simulink model "control_main"  (R2026a)
settings: Solver=VariableStepAuto  StopTime=inf
InitFcn:
  | load(fullfile('calibration_data','sensor_calibration.mat'),'coefficients');
  | load(fullfile('calibration_data','pump_calibration.mat'),'Q');
  | load(fullfile('calibration_data','az_calibration.mat'),'az');
  | 
  | actuallevel1 = 200;
values from neighbouring files (symbols this model uses):
  coefficients = [20.111978783 20.2762923351 20.4770477048]    [sensor_calibration.mat]
  sensor_low = [1.00893772894 1.03633699634 1.00974358974]    [sensor_calibration.mat]
undefined symbols (not defined in the file or in its folder): az, Q
libraries: instrumentseriallib x3
settings Model: Creator=user  LastModifiedBy=jinyu

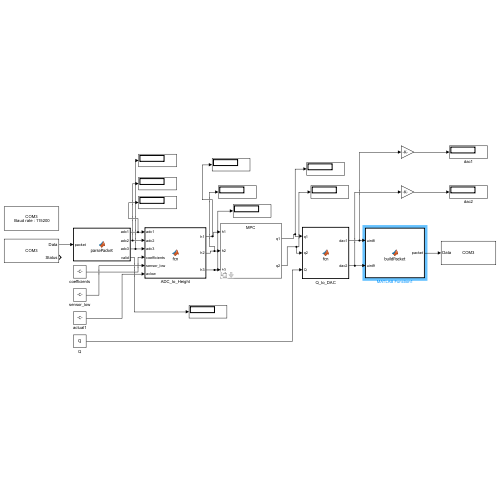
[thumbnail: Simulink's stored preview of the top-level diagram]
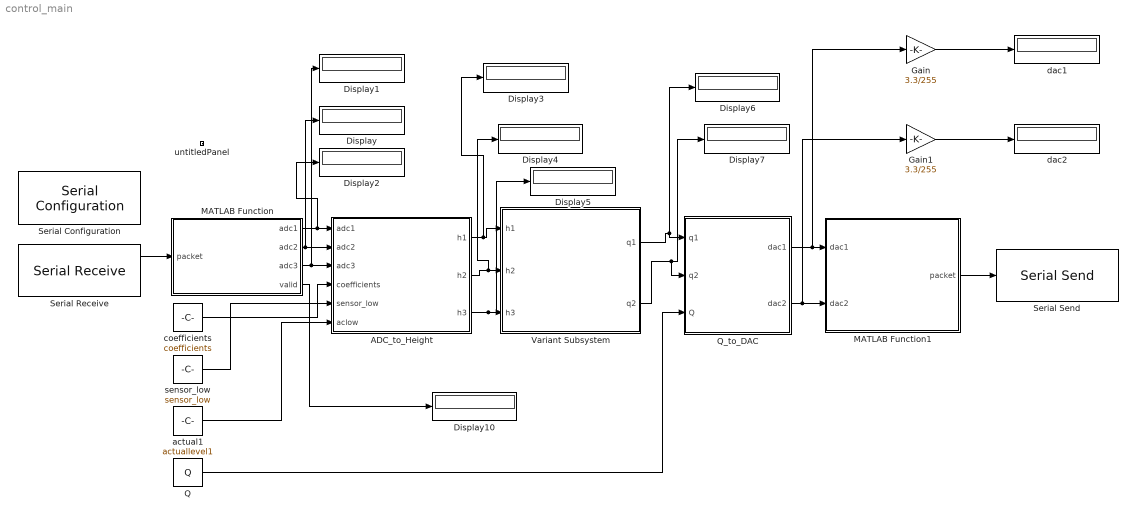
== system control_main ==
  ADC_to_Height : MATLAB Function  TreatAsAtomicUnit=on
  Display{,1..7,10} (9 alike) : Display
  Gain : Gain  Gain=3.3/255
  Gain1 : Gain  Gain=3.3/255
  MATLAB Function : MATLAB Function  TreatAsAtomicUnit=on
  MATLAB Function1 : MATLAB Function  TreatAsAtomicUnit=on
  Q : Constant  Value=Q
  Q_to_DAC : MATLAB Function  TreatAsAtomicUnit=on
  Serial Configuration : instrumentseriallib/Serial Configuration  Priority=-200000  PortSel=COM3  Port=COM3  ComPort=COM3  BaudRate=115200  DataBits=8  Parity=none  StopBits=1  ByteOrder=little-endian  FlowControl=none  Timeout=10  SimulateUsing=Interpreted execution  BlockInModel=on  aMode=1
  Serial Receive : instrumentseriallib/Serial Receive  Priority=1  PortSel=COM3  Port=COM3  ComPort=COM3  DataType=uint8  SaveDataType=uint8  ToggleHeader=on  Header=[0xAA 0x01]  ToggleDataSize=on  DataSize=[7]  ToggleTerminator=off  Terminator=<none>  CustomTerminator=[]  InputFormat=Column major  EnableBlockingMode=off  ActionDataUnavailable=Output last received value  ActionWhenDataUnavailable=Output last received value  CustomValue=0  SampleTime=0.01  SimulateUsing=Interpreted execution  BlockInModel=on  aMode=1  LibraryInUse=instrumentlib
  Serial Send : instrumentseriallib/Serial Send  Priority=1  PortSel=COM3  Port=COM3  ComPort=COM3  Header=[]  Terminator=<none>  CustomTerminator=[]  EnableBlockingMode=off  SimulateUsing=Interpreted execution  BlockInModel=on  aMode=1
  Variant Subsystem : Subsystem  Variant=on  mask{ctrl_mode=MPC, r1=300, r2=150, r3=200, Kp_PI=1, Ki_PI=1, Kp1_PI=1, Ki1_PI=1, Kp2_PI=1, Ki2_PI=1, Kp_IO=1, Kp1_IO=1, Kp3_IO=1, Kd3_IO=1, K_BS=1, Kz_BS=1, K1_BS=1, K3_BS=1, S1=0.05, S2=0.05, S3=20, R1_MPC=0.05, R2_MPC=0.05, H=15}
      mask prompts: r1 "Tank1"; r2 "Tank2"; r3 "Tank3"; Kp_PI "Kp"; Ki_PI "Ki"; Kp1_PI "Kp1"; Ki1_PI "Ki1"; Kp2_PI "Kp2"; Ki2_PI "Ki2"; Kp_IO "Kp"; Kp1_IO "Kp1"; Kp3_IO "Kp3"; Kd3_IO "Kd3"; K_BS "K"; Kz_BS "Kz"; K1_BS "K1"; K3_BS "K3"; R1_MPC "R1"; R2_MPC "R2"
      mask DialogControl ParameterGroupVar Prompt: Controller
      mask DialogControl Container4 Prompt: Reference Levels
      mask DialogControl Container5 Prompt: PI SISO Parameters
      mask DialogControl Container6 Prompt: PI MIMO Parameters
      mask DialogControl Container7 Prompt: IO Linearization SISO
      mask DialogControl Container8 Prompt: IO Linearization MIMO
      mask DialogControl Container9 Prompt: Backstepping SISO
      mask DialogControl Container10 Prompt: Backstepping MIMO
      mask DialogControl Container11 Prompt: MPC
  actual1 : Constant  Value=actuallevel1
  coefficients : Constant  Value=coefficients
  dac1 : Display
  dac2 : Display
  sensor_low : Constant  Value=sensor_low
  untitledPanel : Subsystem  Tag=HiddenForWebPanel  IsWebBlockPanel=on
  wires:
  MATLAB Function1/1(packet) -> Serial Send/1
  Serial Receive/1 -> MATLAB Function/1(packet)
  MATLAB Function/2(adc2) -> ADC_to_Height/2(adc2), Display/1
  MATLAB Function/3(adc3) -> ADC_to_Height/3(adc3), Display1/1
  coefficients/1 -> ADC_to_Height/4(coefficients)
  sensor_low/1 -> ADC_to_Height/5(sensor_low)
  actual1/1 -> ADC_to_Height/6(aclow)
  Q_to_DAC/1(dac1) -> Gain/1, MATLAB Function1/1(dac1)
  Q_to_DAC/2(dac2) -> Gain1/1, MATLAB Function1/2(dac2)
  Q/1 -> Q_to_DAC/3(Q)
  ADC_to_Height/1(h1) -> Display3/1, Variant Subsystem/1(h1)
  ADC_to_Height/2(h2) -> Display4/1, Variant Subsystem/2(h2)
  ADC_to_Height/3(h3) -> Display5/1, Variant Subsystem/3(h3)
  Variant Subsystem/1(q1) -> Display6/1, Q_to_DAC/1(q1)
  Variant Subsystem/2(q2) -> Display7/1, Q_to_DAC/2(q2)
  MATLAB Function/1(adc1) -> ADC_to_Height/1(adc1), Display2/1
  MATLAB Function/4(valid) -> Display10/1
  Gain/1 -> dac1/1
  Gain1/1 -> dac2/1

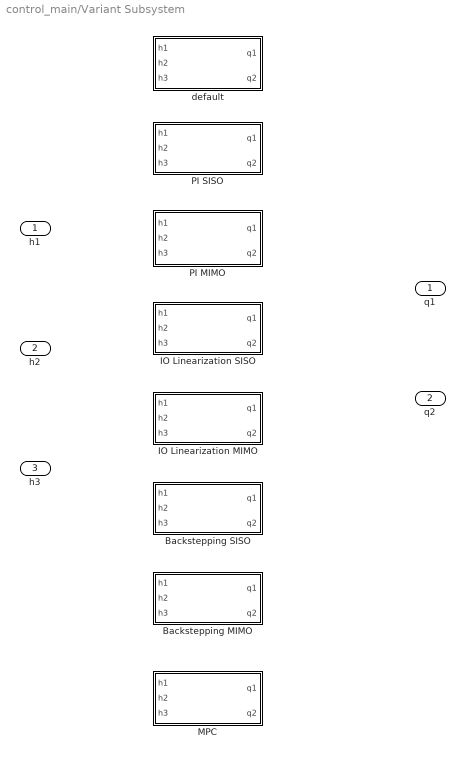
== system control_main/Variant Subsystem ==
  h1 : Inport
  h2 : Inport  Port=2
  h3 : Inport  Port=3
  Backstepping MIMO : Subsystem  VariantControl=ctrl_mode == 6
  Backstepping SISO : Subsystem  VariantControl=ctrl_mode == 5
  IO Linearization MIMO : Subsystem  VariantControl=ctrl_mode == 4
  IO Linearization SISO : Subsystem  VariantControl=ctrl_mode == 3
  MPC : Subsystem  VariantControl=ctrl_mode == 7
  PI MIMO : Subsystem  VariantControl=ctrl_mode == 2
  PI SISO : Subsystem  VariantControl=ctrl_mode == 1
  default : Subsystem  VariantControl=ctrl_mode == 0
  q1 : Outport
  q2 : Outport  Port=2

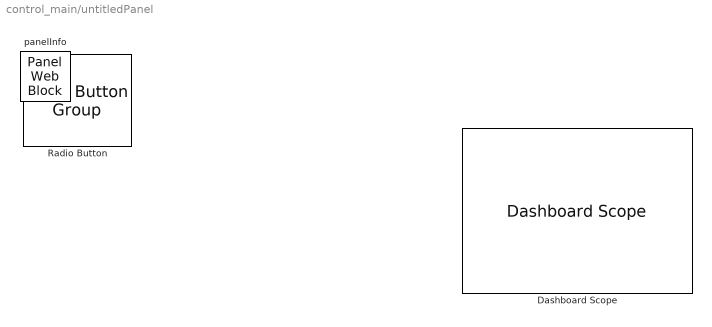
== system control_main/untitledPanel ==
  Dashboard Scope : DashboardScope  Tag=HiddenForWebPanel  PanelInfo="{\"height\":404,\"left\":393,\"panelId\":\"panelId-8aad0df7-f305-4620-9adc-6ae666dad641\",\"top\":27,\"type\":\"panelChild\",\"version\":\"2019b\",\"width\":464,\"zIndex\":1500004}"  Ymin=50  Ymax=550  FontColor=[0.0, 0.0, 0.0]
  Radio Button : RadioButtonGroup  Tag=HiddenForWebPanel  PanelInfo="{\"height\":384,\"left\":33,\"panelId\":\"panelId-8aad0df7-f305-4620-9adc-6ae666dad641\",\"top\":42,\"type\":\"panelChild\",\"version\":\"2019b\",\"width\":318,\"zIndex\":1500002}"  ButtonGroupName=Control Mode
  panelInfo : PanelWebBlock  Tag=HiddenForWebPanel  PanelInfo="{\"compacted\":true,\"height\":468,\"isActiveTab\":true,\"left\":782,\"name\":\"Panel\",\"panelId\":\"panelId-8aad0df7-f305-4620-9adc-6ae666dad641\",\"tabIndex\":0,\"tabbedSetId\":\"tabbedSet3175960063\",\"top\":92,\"type\":\"panel\",\"version\":\"2019b\",\"visible\":true,\"width\":881,\"zIndex\":1500002}"  PanelSnapshot=<binary blob, 100836 chars, not shown>

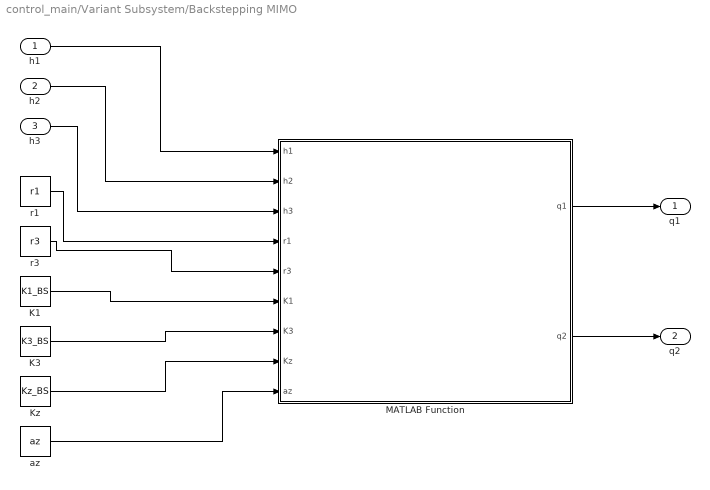
== system control_main/Variant Subsystem/Backstepping MIMO ==
  h1 : Inport
  h2 : Inport  Port=2
  h3 : Inport  Port=3
  K1 : Constant  Value=K1_BS
  K3 : Constant  Value=K3_BS
  Kz : Constant  Value=Kz_BS
  MATLAB Function : MATLAB Function  TreatAsAtomicUnit=on
  az : Constant  Value=az
  r1 : Constant  Value=r1
  r3 : Constant  Value=r3
  q1 : Outport
  q2 : Outport  Port=2
  wires:
  MATLAB Function/1(q1) -> q1/1
  MATLAB Function/2(q2) -> q2/1
  h1/1 -> MATLAB Function/1(h1)
  h2/1 -> MATLAB Function/2(h2)
  h3/1 -> MATLAB Function/3(h3)
  r1/1 -> MATLAB Function/4(r1)
  r3/1 -> MATLAB Function/5(r3)
  K1/1 -> MATLAB Function/6(K1)
  K3/1 -> MATLAB Function/7(K3)
  Kz/1 -> MATLAB Function/8(Kz)
  az/1 -> MATLAB Function/9(az)

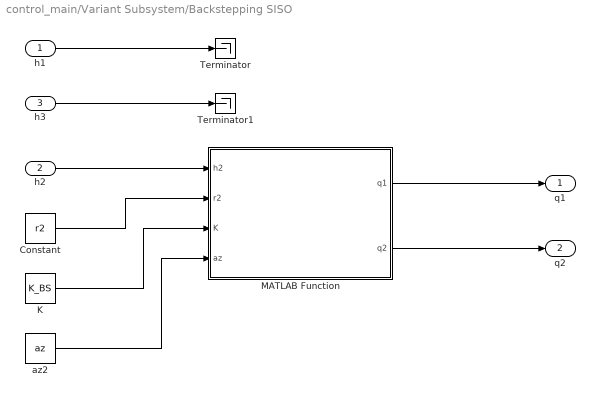
== system control_main/Variant Subsystem/Backstepping SISO ==
  h1 : Inport
  h2 : Inport  Port=2
  h3 : Inport  Port=3
  Constant : Constant  Value=r2
  K : Constant  Value=K_BS
  MATLAB Function : MATLAB Function  TreatAsAtomicUnit=on
  Terminator : Terminator
  Terminator1 : Terminator
  az2 : Constant  Value=az
  q1 : Outport
  q2 : Outport  Port=2
  wires:
  Constant/1 -> MATLAB Function/2(r2)
  az2/1 -> MATLAB Function/4(az)
  MATLAB Function/1(q1) -> q1/1
  MATLAB Function/2(q2) -> q2/1
  K/1 -> MATLAB Function/3(K)
  h3/1 -> Terminator1/1
  h2/1 -> MATLAB Function/1(h2)
  h1/1 -> Terminator/1

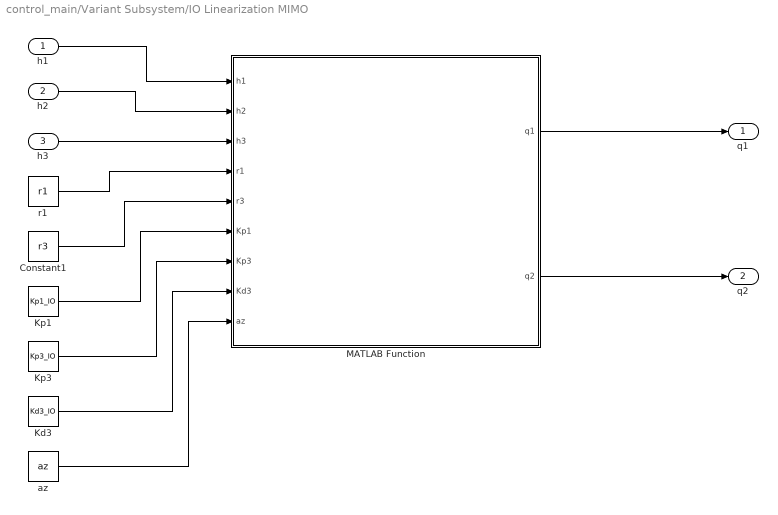
== system control_main/Variant Subsystem/IO Linearization MIMO ==
  h1 : Inport
  h2 : Inport  Port=2
  h3 : Inport  Port=3
  Constant1 : Constant  Value=r3
  Kd3 : Constant  Value=Kd3_IO
  Kp1 : Constant  Value=Kp1_IO
  Kp3 : Constant  Value=Kp3_IO
  MATLAB Function : MATLAB Function  TreatAsAtomicUnit=on
  az : Constant  Value=az
  r1 : Constant  Value=r1
  q1 : Outport
  q2 : Outport  Port=2
  wires:
  h2/1 -> MATLAB Function/2(h2)
  MATLAB Function/2(q2) -> q2/1
  MATLAB Function/1(q1) -> q1/1
  h1/1 -> MATLAB Function/1(h1)
  h3/1 -> MATLAB Function/3(h3)
  r1/1 -> MATLAB Function/4(r1)
  Constant1/1 -> MATLAB Function/5(r3)
  Kp1/1 -> MATLAB Function/6(Kp1)
  Kp3/1 -> MATLAB Function/7(Kp3)
  Kd3/1 -> MATLAB Function/8(Kd3)
  az/1 -> MATLAB Function/9(az)

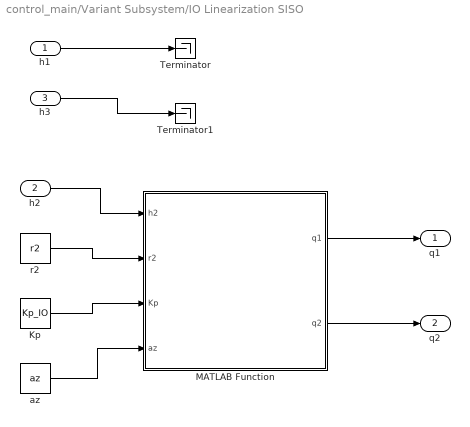
== system control_main/Variant Subsystem/IO Linearization SISO ==
  h1 : Inport
  h2 : Inport  Port=2
  h3 : Inport  Port=3
  Kp : Constant  Value=Kp_IO
  MATLAB Function : MATLAB Function  TreatAsAtomicUnit=on
  Terminator : Terminator
  Terminator1 : Terminator
  az : Constant  Value=az
  r2 : Constant  Value=r2
  q1 : Outport
  q2 : Outport  Port=2
  wires:
  h2/1 -> MATLAB Function/1(h2)
  r2/1 -> MATLAB Function/2(r2)
  Kp/1 -> MATLAB Function/3(Kp)
  MATLAB Function/1(q1) -> q1/1
  MATLAB Function/2(q2) -> q2/1
  az/1 -> MATLAB Function/4(az)
  h1/1 -> Terminator/1
  h3/1 -> Terminator1/1

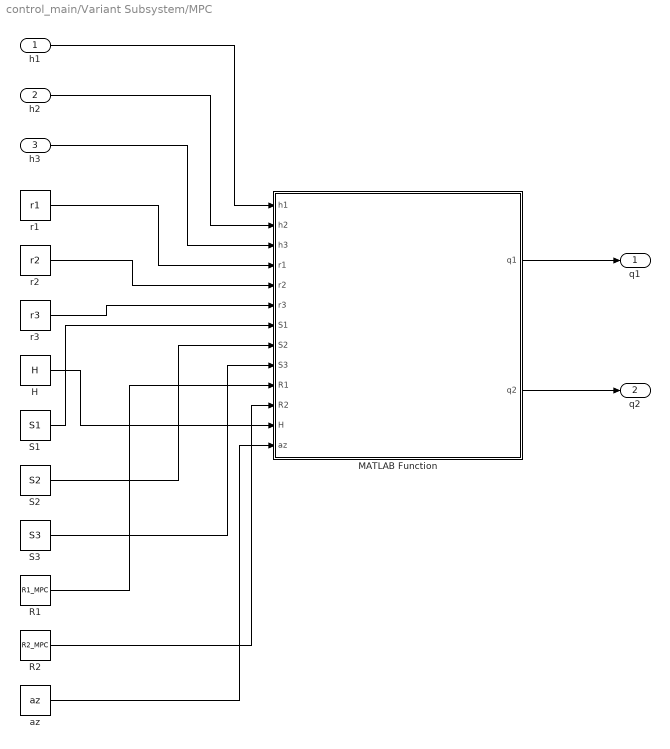
== system control_main/Variant Subsystem/MPC ==
  h1 : Inport
  h2 : Inport  Port=2
  h3 : Inport  Port=3
  H : Constant  Value=H
  MATLAB Function : MATLAB Function  TreatAsAtomicUnit=on
  R1 : Constant  Value=R1_MPC
  R2 : Constant  Value=R2_MPC
  S1 : Constant  Value=S1
  S2 : Constant  Value=S2
  S3 : Constant  Value=S3
  az : Constant  Value=az
  r1 : Constant  Value=r1
  r2 : Constant  Value=r2
  r3 : Constant  Value=r3
  q1 : Outport
  q2 : Outport  Port=2
  wires:
  MATLAB Function/1(q1) -> q1/1
  MATLAB Function/2(q2) -> q2/1
  h1/1 -> MATLAB Function/1(h1)
  h2/1 -> MATLAB Function/2(h2)
  h3/1 -> MATLAB Function/3(h3)
  r1/1 -> MATLAB Function/4(r1)
  r2/1 -> MATLAB Function/5(r2)
  r3/1 -> MATLAB Function/6(r3)
  H/1 -> MATLAB Function/12(H)
  S1/1 -> MATLAB Function/7(S1)
  S2/1 -> MATLAB Function/8(S2)
  S3/1 -> MATLAB Function/9(S3)
  R1/1 -> MATLAB Function/10(R1)
  R2/1 -> MATLAB Function/11(R2)
  az/1 -> MATLAB Function/13(az)

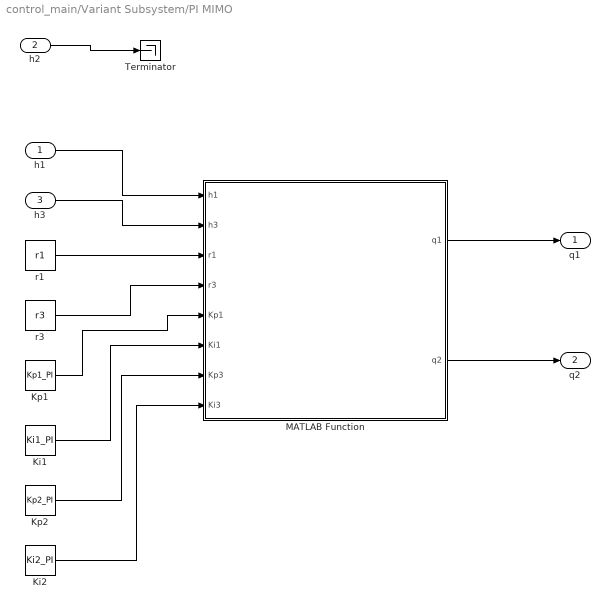
== system control_main/Variant Subsystem/PI MIMO ==
  h1 : Inport
  h2 : Inport  Port=2
  h3 : Inport  Port=3
  Ki1 : Constant  Value=Ki1_PI
  Ki2 : Constant  Value=Ki2_PI
  Kp1 : Constant  Value=Kp1_PI
  Kp2 : Constant  Value=Kp2_PI
  MATLAB Function : MATLAB Function  TreatAsAtomicUnit=on
  Terminator : Terminator
  r1 : Constant  Value=r1
  r3 : Constant  Value=r3
  q1 : Outport
  q2 : Outport  Port=2
  wires:
  MATLAB Function/2(q2) -> q2/1
  MATLAB Function/1(q1) -> q1/1
  h1/1 -> MATLAB Function/1(h1)
  h3/1 -> MATLAB Function/2(h3)
  r1/1 -> MATLAB Function/3(r1)
  r3/1 -> MATLAB Function/4(r3)
  Kp1/1 -> MATLAB Function/5(Kp1)
  Ki1/1 -> MATLAB Function/6(Ki1)
  Kp2/1 -> MATLAB Function/7(Kp3)
  Ki2/1 -> MATLAB Function/8(Ki3)
  h2/1 -> Terminator/1

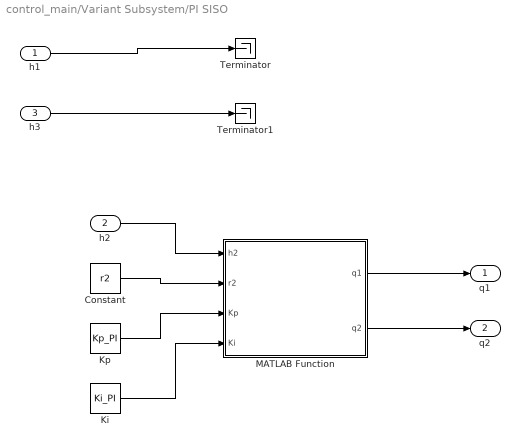
== system control_main/Variant Subsystem/PI SISO ==
  h1 : Inport
  h2 : Inport  Port=2
  h3 : Inport  Port=3
  Constant : Constant  Value=r2
  Ki : Constant  Value=Ki_PI
  Kp : Constant  Value=Kp_PI
  MATLAB Function : MATLAB Function  TreatAsAtomicUnit=on
  Terminator : Terminator
  Terminator1 : Terminator
  q1 : Outport
  q2 : Outport  Port=2
  wires:
  MATLAB Function/2(q2) -> q2/1
  MATLAB Function/1(q1) -> q1/1
  h2/1 -> MATLAB Function/1(h2)
  Constant/1 -> MATLAB Function/2(r2)
  Kp/1 -> MATLAB Function/3(Kp)
  Ki/1 -> MATLAB Function/4(Ki)
  h1/1 -> Terminator/1
  h3/1 -> Terminator1/1

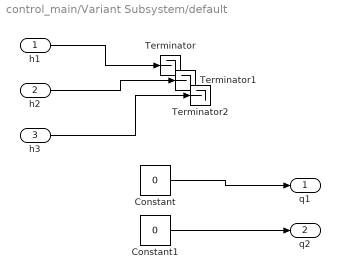
== system control_main/Variant Subsystem/default ==
  h1 : Inport
  h2 : Inport  Port=2
  h3 : Inport  Port=3
  Constant : Constant  Value=0
  Constant1 : Constant  Value=0
  Terminator : Terminator
  Terminator1 : Terminator
  Terminator2 : Terminator
  q1 : Outport
  q2 : Outport  Port=2
  wires:
  Constant/1 -> q1/1
  Constant1/1 -> q2/1
  h1/1 -> Terminator/1
  h2/1 -> Terminator1/1
  h3/1 -> Terminator2/1

== matlab function control_main/Variant Subsystem/IO Linearization MIMO/MATLAB Function ==
  data: h1 input; q1 output; h2 input; h3 input; r1 input; r3 input; Kp1 input; Kp3 input; Kd3 input; az input; q2 output
function [q1,q2] = IO_MIMO(h1,h2,h3,r1,r3,Kp1,Kp3,Kd3,az)
%对q13和q32分别求一阶和二阶导推q1q2表达式

A  = 154.0;
Sn = 0.5;
g  = 981.0;
TWOG = 2*g;

az1 = az(1);
az2 = az(2);
az3 = az(3);

q13 = az1 * Sn * sqrt(TWOG * abs(h1-h3));
q32 = az3 * Sn * sqrt(TWOG * abs(h3-h2));
q20 = az2 * Sn * sqrt(TWOG * max(h2,0));

e1 = r1 - h1;
q1 = A*Kp1*e1 + 2*q13 - q32;
q1 = min(max(q1,0),800);

den13 = sqrt(abs(h1-h3));
den32 = sqrt(abs(h3-h2));

if den13 < 1e-6
    den13 = 1e-6;
end

if den32 < 1e-6
    den32 = 1e-6;
end

k1 = az1 * den32 / (az3 * den13);
k2 = (TWOG * az3 * Sn) / (2 * sqrt(TWOG * abs(h3-h2) + 1e-6));

persistent e3_old

if isempty(e3_old)
    e3_old = 0;
end

Ts = 0.01;
e3 = r3 - h3;

pd = Kp3*e3 + Kd3*(e3 - e3_old)/Ts;

q2 = -k1*(q1 - 2*q13 + q32) ...
     + (q13 - 2*q32 + q20) ...
     + A*A*(1/k2)*pd;

q2 = min(max(q2,0),800);

e3_old = e3;

end

== matlab function control_main/Variant Subsystem/Backstepping SISO/MATLAB Function ==
  data: h2 input; q1 output; r2 input; K input; az input; q2 output
function [q1,q2] = Backstepping_SISO(h2,r2,K,az)
% backstepping误差指数减小  de/dt=-Ke​

A  = 154.0;
Sn = 0.5;
g  = 981.0;
Ofc2 = az(2);

q20 = Ofc2 * Sn * sqrt(2*g*max(h2,0));

q1 = 0;
q2 = q20 + A*K*(r2 - h2);

q2 = min(max(q2,0),800);

end

== matlab function control_main/Variant Subsystem/Backstepping MIMO/MATLAB Function ==
  data: h1 input; q1 output; h2 input; h3 input; r1 input; r3 input; K1 input; K3 input; Kz input; az input; q2 output
function [q1,q2] = Backstepping_MIMO(h1,h2,h3,r1,r3,K1,K3,Kz,az)
% Backstepping MIMO for Tank1 and Tank3
% K1       : Tank1 error gain
% K3       : Tank3 virtual control gain
% Kz       : q32 tracking gain


A  = 154.0;
Sn = 0.5;
g  = 981.0;
TWOG = 2*g;
epsv = 1e-6;

az1 = az(1);
az2 = az(2);
az3 = az(3);

q13 = az1 * Sn * sqrt(TWOG * max(h1-h3, 0));
q32 = az3 * Sn * sqrt(TWOG * max(h3-h2, 0));
q20 = az2 * Sn * sqrt(TWOG * max(h2,    0));

if r1 == 0 && r3 == 0
    q1 = 0;
    q2 = 0;
    return;
else
end
% Step 1: control h1
% e1 = h1 - r1, desired e1_dot = -K1*e1
% q1 = q13 - A*K1*e1

e1 = h1 - r1;

q1 = q13 - A*K1*e1;
q1 = min(max(q1,0),800);

% Step 2: virtual control for h3
% e3 = h3 - r3
% desired e3_dot = -K3*e3
% q32_des = q13 + A*K3*e3
e3 = h3 - r3;

q32_des = q13 + A*K3*e3;

% virtual tracking error
z = q32 - q32_des;

% Compute derivative of q32_des
% q32_des_dot = q13_dot + A*K3*e3_dot
% e3_dot = h3_dot = (q13-q32)/A
% q13_dot = k13*(h1_dot-h3_dot)
dh13 = max(h1-h3, epsv);
dh32 = max(h3-h2, epsv);

k13 = (az1 * Sn * TWOG) / (2 * sqrt(TWOG * dh13));
k32 = (az3 * Sn * TWOG) / (2 * sqrt(TWOG * dh32));

h1_dot = (q1 - q13) / A;
h3_dot = (q13 - q32) / A;

q13_dot = k13 * (h1_dot - h3_dot);

q32_des_dot = q13_dot + A*K3*h3_dot;

% Step 3: real control q2
% z_dot = -Kz*z
%
% q2 = q13 - 2*q32 + q20
%      - (A/k32)*q32_des_dot
%      + (A/k32)*Kz*z
q2 = q13 - 2*q32 + q20 ...
     - (A/k32)*q32_des_dot ...
     + (A/k32)*Kz*z;

q2 = min(max(q2,0),800);

end

== matlab function control_main/Variant Subsystem/MPC/MATLAB Function ==
  data: h1 input; q1 output; h2 input; h3 input; r1 input; r2 input; r3 input; S1 input; S2 input; S3 input; R1 input; R2 input; H input; az input; q2 output
function [q1,q2] = MPC(h1,h2,h3,r1,r2,r3,S1,S2,S3,R1,R2,H,az)
%#codegen

A  = 154.0;
Sn = 0.5;
g  = 981.0;
Ts = 0.1;
Qmax = 800.0;

H = round(H);
if H < 1
    H = 1;
end
if H > 20
    H = 20;
end

az1 = az(1);
az2 = az(2);
az3 = az(3);

C1 = az1 * Sn;
C2 = az3 * Sn;
C3 = az2 * Sn;

x = [h1; h2; h3];
r = [r1; r2; r3];

x0 = max(r,0.1);
u0 = steadyInput(x0,C1,C2,C3,g);

[Ad,Bd] = linearModel(x0,Ts,A,C1,C2,C3,g);

nx = 3;
nu = 2;
ny = 3;
Hmax = 20;

Phi   = zeros(ny*Hmax,nx);
Gamma = zeros(ny*Hmax,nu*Hmax);

for i = 1:Hmax
    Ai = eye(nx);

    for k = 1:i
        Ai = Ai * Ad;
    end

    if i <= H
        Phi((i-1)*ny+1:i*ny,:) = Ai;
    end

    for j = 1:Hmax
        if j <= i && i <= H && j <= H
            Aij = eye(nx);

            for k = 1:(i-j)
                Aij = Aij * Ad;
            end

            Gamma((i-1)*ny+1:i*ny,(j-1)*nu+1:j*nu) = Aij * Bd;
        end
    end
end

Sbar = zeros(ny*Hmax,ny*Hmax);
Rbar = zeros(nu*Hmax,nu*Hmax);

S = diag([S1 S2 S3]);
R = diag([R1 R2]);

for i = 1:Hmax
    if i <= H
        Sbar((i-1)*ny+1:i*ny,(i-1)*ny+1:i*ny) = S;
        Rbar((i-1)*nu+1:i*nu,(i-1)*nu+1:i*nu) = R;
    else
        Sbar((i-1)*ny+1:i*ny,(i-1)*ny+1:i*ny) = eye(ny);
        Rbar((i-1)*nu+1:i*nu,(i-1)*nu+1:i*nu) = 1e6 * eye(nu);
    end
end

Rref  = zeros(ny*Hmax,1);
X0ref = zeros(ny*Hmax,1);

for i = 1:Hmax
    if i <= H
        Rref((i-1)*ny+1:i*ny)  = r;
        X0ref((i-1)*ny+1:i*ny) = x0;
    else
        Rref((i-1)*ny+1:i*ny)  = x0;
        X0ref((i-1)*ny+1:i*ny) = x0;
    end
end

dx0 = x - x0;

G = Gamma' * Sbar * Gamma + Rbar;
F = Gamma' * Sbar * (X0ref + Phi*dx0 - Rref);

dU = -G \ F;

u = u0 + dU(1:2);
% Fnorm = norm(F);
% dUnorm = norm(dU);

q1 = min(max(u(1),0),Qmax);
q2 = min(max(u(2),0),Qmax);

end

function [Ad,Bd] = linearModel(x0,Ts,A,C1,C2,C3,g)

epsv = 1e-6;

h1 = max(x0(1),0);
h2 = max(x0(2),0);
h3 = max(x0(3),0);

d13 = h1 - h3;
d32 = h3 - h2;

if abs(d13) < epsv
    d13 = epsv;
end

if abs(d32) < epsv
    d32 = epsv;
end

k13 = C1 * g / sqrt(2*g*abs(d13));
k32 = C2 * g / sqrt(2*g*abs(d32));
k20 = C3 * g / sqrt(2*g*max(h2,epsv));

Ac = zeros(3,3);

Ac(1,1) = -k13/A;
Ac(1,3) =  k13/A;

Ac(2,2) = (-k32 - k20)/A;
Ac(2,3) =  k32/A;

Ac(3,1) =  k13/A;
Ac(3,2) =  k32/A;
Ac(3,3) = (-k13 - k32)/A;

Bc = [1/A 0;
      0   1/A;
      0   0];

Ad = eye(3) + Ts * Ac;
Bd = Ts * Bc;

end

function u0 = steadyInput(x,C1,C2,C3,g)

h1 = max(x(1),0);
h2 = max(x(2),0);
h3 = max(x(3),0);

q13 = C1 * sign(h1-h3) * sqrt(2*g*abs(h1-h3));
q32 = C2 * sign(h3-h2) * sqrt(2*g*abs(h3-h2));
q20 = C3 * sqrt(2*g*h2);

u0 = zeros(2,1);
u0(1) = q13;
u0(2) = q20 - q32;

u0 = max(u0,0);

end

== matlab function control_main/MATLAB Function1 ==
  data: dac1 input; packet output; dac2 input
function packet = buildPacket(dac1, dac2)

dac1 = uint8(0);
dac2 = uint8(0);

packet = uint8(zeros(5,1));
packet(1) = hex2dec('BB');
packet(2) = hex2dec('02');
packet(3) = dac1;
packet(4) = dac2;

checksum = uint8(0);
for i = 1:4
    checksum = bitxor(checksum, packet(i));
end
packet(5) = checksum;

== matlab function control_main/MATLAB Function ==
  data: packet input; adc1 output; adc2 output; adc3 output; valid output
function [adc1, adc2, adc3, valid] = parsePacket(packet)

checksum = uint8(0);
for i = 1:6
    checksum = bitxor(checksum, uint8(packet(i)));
end

if checksum == uint8(packet(7))
    adc1 = double(bitshift(uint16(packet(1)), 8) + uint16(packet(2))) * (3.3 / 4095);
    adc2 = double(bitshift(uint16(packet(3)), 8) + uint16(packet(4))) * (3.3 / 4095);
    adc3 = double(bitshift(uint16(packet(5)), 8) + uint16(packet(6))) * (3.3 / 4095);
    valid = true;
else
    adc1 = 0;
    adc2 = 0;
    adc3 = 0;
    valid = false;
end

end

== matlab function control_main/ADC_to_Height ==
  data: adc1 input; h1 output; adc2 input; adc3 input; coefficients input; sensor_low input; aclow input; h2 output; h3 output
function [h1,h2,h3] = fcn(adc1,adc2,adc3,coefficients,sensor_low,aclow)

h1 = coefficients(1) * (adc1 - sensor_low(1)) + aclow;
h2 = coefficients(3) * (adc3 - sensor_low(3)) + aclow;
h3 = coefficients(2) * (adc2 - sensor_low(2)) + aclow;

end

== matlab function control_main/Q_to_DAC ==
  data: q1 input; dac1 output; q2 input; Q input; dac2 output
function [dac1,dac2] = fcn(q1,q2,Q)

dac_table = [255 223 191 159 128 96 64 32 0];

q1 = min(max(q1, Q(1,1)), Q(1,end));
q2 = min(max(q2, Q(2,1)), Q(2,end));

dac1 = interp1(Q(1,:), dac_table, q1, 'linear');
dac2 = interp1(Q(2,:), dac_table, q2, 'linear');

dac1 = min(max(dac1,0),255);
dac2 = min(max(dac2,0),255);

end

== matlab function control_main/Variant Subsystem/PI MIMO/MATLAB Function ==
  data: h1 input; h3 input; r1 input; r3 input; Kp1 input; Ki1 input; q1 output; Kp3 input; Ki3 input; q2 output
function [q1, q2] = PI_MIMO_T1T3(h1, h3, r1, r3, Kp1, Ki1, Kp3, Ki3)
%#codegen

persistent q1_old e1_old
persistent q2_old e3_old

if isempty(q1_old)
    q1_old = 0;
    e1_old = 0;
    q2_old = 0;
    e3_old = 0;
end

Ts = 0.01;

% PI loop 1: h1 -> q1
e1 = r1 - h1;
k1 = Ki1 * Ts / 2;
zk10 = Kp1 + k1;
zk11 = k1 - Kp1;

q1_new = q1_old + zk10 * e1 + zk11 * e1_old;
q1_new = min(max(q1_new, 0), 800);

% PI loop 2: h3 -> q2
e3 = r3 - h3;
k3 = Ki3 * Ts / 2;
zk30 = Kp3 + k3;
zk31 = k3 - Kp3;

q2_new = q2_old + zk30 * e3 + zk31 * e3_old;
q2_new = min(max(q2_new, 0), 800);

q1 = q1_new;
q2 = q2_new;

q1_old = q1_new;
e1_old = e1;

q2_old = q2_new;
e3_old = e3;

end

== matlab function control_main/Variant Subsystem/PI SISO/MATLAB Function ==
  data: h2 input; q1 output; r2 input; Kp input; Ki input; q2 output
function [q1,q2] = PI_SISO(h2,r2,Kp,Ki)

persistent u_old e_old

if isempty(u_old)
    u_old = 0;
    e_old = 0;
end

% ESP32 sample time: 100 Hz = 0.01 s
Ts = 0.01;

e = r2 - h2;

k = Ki * Ts / 2;
zk0 = Kp + k;
zk1 = k - Kp;

u = u_old + zk0 * e + zk1 * e_old;

u = min(max(u, 0), 800);

q1 = 0;
q2 = u;

u_old = u;
e_old = e;

end

== matlab function control_main/Variant Subsystem/IO Linearization SISO/MATLAB Function ==
  data: h2 input; q1 output; r2 input; Kp input; az input; q2 output
function [q1,q2] = IO_SISO(h2,r2,Kp,az)

A  = 154;
Sn = 0.5;
g  = 981;

Ofc2 = az(2);

e = r2 - h2;

% IO linearization
q1 = 0;
q2 = A*Kp*e + Ofc2*Sn*sqrt(2*g*max(h2,0));

q2 = min(max(q2,0),800);

end
